simulink model "RefBlocks"  (R2020b)
settings: Solver=VariableStepAuto  StartTime=0.0  StopTime=10.0  RelTol=1e-3
values from neighbouring files (symbols this model uses):
  accel = 10000    [init_sim.m]
  Bm = 0    [init_sim.m]
  Ctrl_type = 3    [init_sim.m]
  dT = motorModel.SyreDrive.Converter.dT * 1e-6    [init_sim.m]
  expC = motorModel.IronPMLossMap_dq.expC    [init_sim.m]
  expH = motorModel.IronPMLossMap_dq.expH    [init_sim.m]
  expPM = motorModel.IronPMLossMap_dq.expPM    [init_sim.m]
  fD_pu_norm = motorModel.FluxMapInv_dq.fD_pu_norm    [init_sim.m]
  fD_vct_max = motorModel.FluxMapInv_dq.fD_vct_max    [init_sim.m]
  fD_vct_ref = motorModel.FluxMapInv_dq.fD_vct_ref    [init_sim.m]
  Fm = interp2(Idd,Iqq,Fdd,0,0)    [init_sim.m]
  fQ_pu_norm = motorModel.FluxMapInv_dq.fQ_pu_norm    [init_sim.m]
  fQ_vct_max = motorModel.FluxMapInv_dq.fQ_vct_max    [init_sim.m]
  fQ_vct_ref = motorModel.FluxMapInv_dq.fQ_vct_ref    [init_sim.m]
  Id_dqt = interpn(motorModel.FluxMapInv_dqt.dataF.Fd,motorModel.FluxMapInv_dqt.dataF.Fq,motorModel.FluxMapInv_dqt.dataF.th,motorModel.FluxMapInv_dqt.dataF.Id,Fd_dqt,Fq_dqt,th_dqt,'cubic')    [init_sim.m]
  Id_fe = motorModel.IronPMLossMap_dq.Id    [init_sim.m]
  id_MTPA = interp1(abs(MTPA.id+1i*MTPA.iq),MTPA.id,i0)    [init_sim.m]
  iD_pu_norm = motorModel.FluxMapInv_dq.iD_pu_norm    [init_sim.m]
  Iq_dqt = interpn(motorModel.FluxMapInv_dqt.dataF.Fd,motorModel.FluxMapInv_dqt.dataF.Fq,motorModel.FluxMapInv_dqt.dataF.th,motorModel.FluxMapInv_dqt.dataF.Iq,Fd_dqt,Fq_dqt,th_dqt,'cubic')    [init_sim.m]
  Iq_fe = motorModel.IronPMLossMap_dq.Iq    [init_sim.m]
  iq_MTPA = interp1(abs(MTPA.id+1i*MTPA.iq),MTPA.iq,i0)    [init_sim.m]
  iQ_pu_norm = motorModel.FluxMapInv_dq.iQ_pu_norm    [init_sim.m]
  IronLoss = 1    [init_sim.m]
  J = motorModel.data.J    [init_sim.m]
  L_sigma = Lq_inic*0.1    [init_sim.m]
  n0 = motorModel.IronPMLossMap_dq.n0    [init_sim.m]
  n_phase = n_set*3    [init_sim.m]
  p = motorModel.data.p    [init_sim.m]
  Pfe_c = motorModel.IronPMLossMap_dq.Pfes_c + motorModel.IronPMLossMap_dq.Pfer_c    [init_sim.m]
  Pfe_h = motorModel.IronPMLossMap_dq.Pfes_h + motorModel.IronPMLossMap_dq.Pfer_h    [init_sim.m]
  Ppm = motorModel.IronPMLossMap_dq.Ppm    [init_sim.m]
  Quad_Maps = 2    [init_sim.m]
  T_dqt = interpn(motorModel.FluxMapInv_dqt.dataF.Fd,motorModel.FluxMapInv_dqt.dataF.Fq,motorModel.FluxMapInv_dqt.dataF.th,motorModel.FluxMapInv_dqt.dataF.T,Fd_dqt,Fq_dqt,th_dqt,'cubic')    [init_sim.m]
  Tf = 0    [init_sim.m]
  th0 = 0    [init_sim.m]
  th_max = max(motorModel.FluxMapInv_dqt.dataF.th,[],'all')    [init_sim.m]
  th_min = min(motorModel.FluxMapInv_dqt.dataF.th,[],'all')    [init_sim.m]
  Ts = 1/motorModel.SyreDrive.Converter.fPWM    [init_sim.m]
  Tv = 0    [init_sim.m]
  VDC = motorModel.data.Vdc    [init_sim.m]
undefined symbols (not defined in the file or in its folder): magnitude, sigbuilder_block, T0
libraries: nesl_utility x8, simulink x4, ee_lib x4, fl_lib x2
(part 1 of 2)
settings Model: Creator=andyb  LastModifiedBy=andyb
settings DebuggingCC: UnconnectedInputMsg=none  UnconnectedOutputMsg=none  UnconnectedLineMsg=none
settings ModelReferenceCC: EnableRefExpFcnMdlSchedulingChecks=off

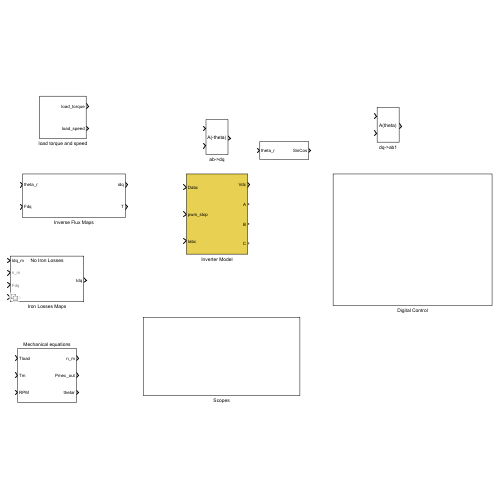
[thumbnail: Simulink's stored preview of the top-level diagram]
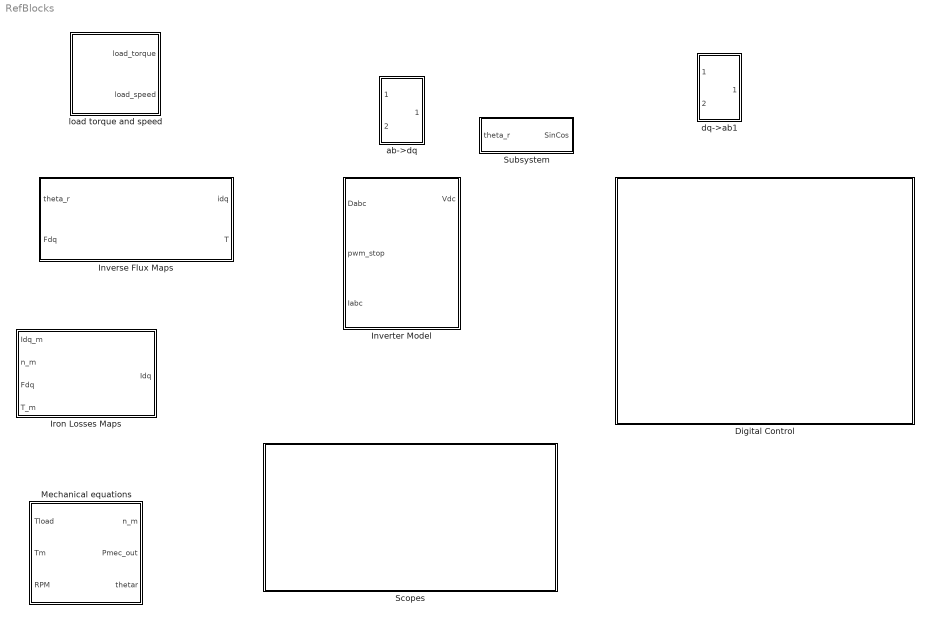
== system RefBlocks ==
  Digital Control : Subsystem
  Inverse Flux Maps : Subsystem
  Inverter Model : Subsystem
  Iron Losses Maps : Subsystem  Variant=on
  Mechanical equations : Subsystem
  Scopes : Subsystem
  Subsystem : Subsystem
  ab->dq : Subsystem
      mask Display: disp('A(-theta)')
  dq->ab1 : Subsystem
      mask Display: disp('A(theta)')
  load torque and speed : Subsystem

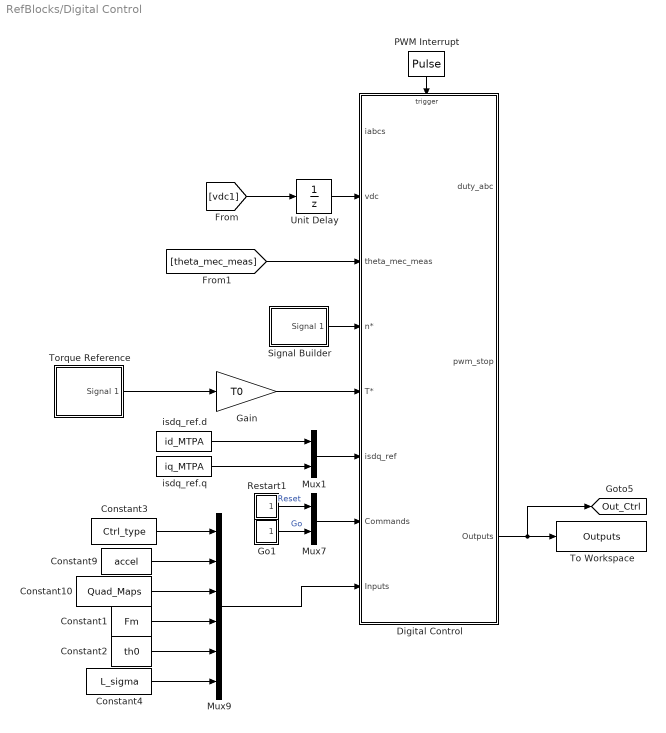
== system RefBlocks/Digital Control ==
  Constant1 : Constant  Value=Fm
  Constant10 : Constant  Value=Quad_Maps
  Constant2 : Constant  Value=th0
  Constant3 : Constant  Value=Ctrl_type
  Constant4 : Constant  Value=L_sigma
  Constant9 : Constant  Value=accel
  Digital Control : Subsystem  TreatAsAtomicUnit=on
  Gain : Gain  Gain=T0
  Go1 : Subsystem
  Mux1 : Mux  Inputs=2
  Mux7 : Mux  Inputs=2
  Mux9 : Mux  Inputs=6
  PWM Interrupt : DiscretePulseGenerator  PulseType=Time based  Period=Ts  PulseWidth=50
  Restart1 : Subsystem
  Signal Builder : Subsystem  Tag=STV Subsys  LoadFcn=sigbuilder_block('load');  StartFcn=sigbuilder_block('start');  StopFcn=sigbuilder_block('stop');  ClipboardFcn=sigbuilder_block('clipboard');  mask(Sigbuilder block){tuvar=[0:10]}
      mask help: Simulink:masks:SigbuilderBlock_MD
      mask init:
      | if ~strcmp(get_param(bdroot(gcbh),'SimulationStatus'),'stopped') tuvar = sigbuilder_block('maskInit'); end
      settings: CopyFcn=sigbuilder_block('copy');  DeleteFcn=sigbuilder_block('delete');  ModelCloseFcn=sigbuilder_block('modelClose');  PreSaveFcn=sigbuilder_block('preSave');  PauseFcn=sigbuilder_block('pause');  ContinueFcn=sigbuilder_block('continue');  NameChangeFcn=sigbuilder_block('namechange');  OpenFcn=sigbuilder_block('open',[163.8 121.8 550.2 399.6 ]);  CloseFcn=sigbuilder_block('close');
      mask Display: plot(0, 0, 100, 100,[2, 2, 32, 32, 2], [68, 8, 8, 68, 68],[32, 2], [38, 38], [32, 19, 2],[53, 60, 44], [32, 17, 17, 2],[16, 16, 31, 31]);txt = getActiveGroup(gcbh);text(2, 100, txt,'verticalAlignment', 'top');
  To Workspace : ToWorkspace  VariableName=Outputs  SaveFormat=Timeseries  SampleTime=-1
  Torque Reference : Subsystem  Tag=STV Subsys  LoadFcn=sigbuilder_block('load');  StartFcn=sigbuilder_block('start');  StopFcn=sigbuilder_block('stop');  ClipboardFcn=sigbuilder_block('clipboard');  mask(Sigbuilder block){tuvar=[0:10]}
      mask help: Simulink:masks:SigbuilderBlock_MD
      mask init:
      | if ~strcmp(get_param(bdroot(gcbh),'SimulationStatus'),'stopped') tuvar = sigbuilder_block('maskInit'); end
      settings: CopyFcn=sigbuilder_block('copy');  DeleteFcn=sigbuilder_block('delete');  ModelCloseFcn=sigbuilder_block('modelClose');  PreSaveFcn=sigbuilder_block('preSave');  PauseFcn=sigbuilder_block('pause');  ContinueFcn=sigbuilder_block('continue');  NameChangeFcn=sigbuilder_block('namechange');  OpenFcn=sigbuilder_block('open',[596.4 129.6 550.2 321.6 ]);  CloseFcn=sigbuilder_block('close');
      mask Display: plot(0, 0, 100, 100,[2, 2, 32, 32, 2], [68, 8, 8, 68, 68],[32, 2], [38, 38], [32, 19, 2],[53, 60, 44], [32, 17, 17, 2],[16, 16, 31, 31]);txt = getActiveGroup(gcbh);text(2, 100, txt,'verticalAlignment', 'top');
  Unit Delay : UnitDelay  SampleTime=-1  HasFrameUpgradeWarning=on
  isdq_ref.d : Constant  Value=id_MTPA
  isdq_ref.q : Constant  Value=iq_MTPA
  tag scope: Out_Ctrl=global
  wires:
  isdq_ref.d/1 -> Mux1/1
  Restart1/1(Res) -> Mux7/1  "Reset"
  Mux9/1 -> Digital Control/8(Inputs)
  PWM Interrupt/1 -> Digital Control/Trigger
  Mux7/1 -> Digital Control/7(Commands)
  Unit Delay/1 -> Digital Control/2(vdc)
  Gain/1 -> Digital Control/5(T*)
  Go1/1(Go) -> Mux7/2  "Go"
  Digital Control/3(Outputs) -> [Out_Ctrl], To Workspace/1
  Constant3/1 -> Mux9/1
  Mux1/1 -> Digital Control/6(isdq_ref)
  Torque Reference/1(Signal 1) -> Gain/1
  Signal Builder/1(Signal 1) -> Digital Control/4(n*)
  isdq_ref.q/1 -> Mux1/2
  [vdc1] -> Unit Delay/1
  [theta_mec_meas] -> Digital Control/3(theta_mec_meas)
  Constant9/1 -> Mux9/2
  Constant10/1 -> Mux9/3
  Constant1/1 -> Mux9/4
  Constant2/1 -> Mux9/5
  Constant4/1 -> Mux9/6

== system RefBlocks/Inverse Flux Maps ==
  theta_r : Inport
  Fdq : Inport  Port=2
  Gain : Gain  Gain=p
  "Inverse Flux Maps " : Subsystem  Variant=on
  idq : Outport
  T : Outport  Port=2
  wires:
  "Inverse Flux Maps "/2(T) -> T/1
  "Inverse Flux Maps "/1(idq) -> idq/1
  theta_r/1 -> Gain/1
  Fdq/1 -> "Inverse Flux Maps "/1(Fdq)
  Gain/1 -> "Inverse Flux Maps "/2(theta_elt)

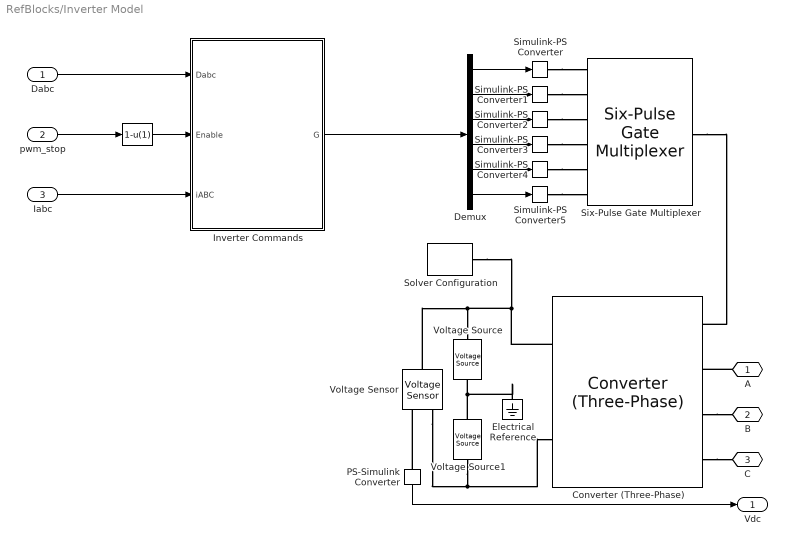
== system RefBlocks/Inverter Model ==
  Dabc : Inport
  pwm_stop : Inport  Port=2
  Iabc : Inport  Port=3
  " " : Fcn  Expr=1-u(1)
  Converter (Three-Phase) : ee_lib/Semiconductors & Converters/Converters/Converter (Three-Phase)  port_option=ee.enum.threePhasePort.expanded  device_type=ee.enum.converters.switchingdevice.ideal  K=0  Vf=0.001 V  Ron=Rd Ohm  Rds=0.001 Ohm  Goff=1e-4 1/Ohm  Vgt=1 V  Vgt_off=-1 V  Ih=1 A  Vth=0.001 V  diode_param=ee.enum.converters.protectiondiode.nodynamics  diode_Vf=0.8 V  diode_Ron=1e-4 Ohm  diode_Goff=1e-5 1/Ohm  diode_C=50 nF  diode_iRM=-235 A  diode_iF=300 A  diode_idot=-50 A/us  diode_trr_param=ee.enum.converters.diodetrr.trr_factor  diode_trr_factor=3  diode_trr=15 us  diode_Qrr=1500 s*uA  snubber_type=ee.enum.converters.snubber.exclude  Cs=1e-7 F  Rs=0.1 Ohm
      settings: InternalSimscapePortConfiguration="{\"Bottom\":[],\"Left\":[{\"id\":\"G\",\"label\":\"G\",\"type\":\"foundation.electrical.twelve_phase\"},{\"id\":\"a\",\"label\":\"a\",\"type\":\"foundation.electrical.electrical\"},{\"id\":\"b\",\"label\":\"b\",\"type\":\"foundation.electrical.electrical\"},{\"id\":\"c\",\"label\":\"c\",\"type\":\"foundation.electrical.electrical\"}],\"Right\":[{\"id\":\"p\",\"label\":\"+\",\"type\":\"foundation.electrical.electrical\"},{\"id\":\"n\",\"label\":\"-\",\"type\":\"foundation.electrical.electrical\"}],\"Top\":[]}"
  Demux : Demux  Outputs=6
  Electrical Reference : fl_lib/Electrical/Electrical Elements/Electrical Reference
  Inverter Commands : Subsystem  Variant=on
  PS-Simulink Converter : nesl_utility/PS-Simulink Converter  PhysicalDomain=network_engine_domain  SubClassName=ps_output  LeftPortType=input  RightPortType=output  PseudoPeriodic=off  Frequencies=[]  VectorFormat=1-D array  Unit=inherit  AffineConversion=off
  Simulink-PS Converter{,1..5} (6 alike) : nesl_utility/Simulink-PS Converter  PhysicalDomain=network_engine_domain  SubClassName=ps_input  LeftPortType=input  RightPortType=output  PseudoPeriodic=off  Frequencies=[]  NoiseDistribution=none  NoiseParameters=[]  Unit=1  AffineConversion=off  FilteringAndDerivatives=provide  SimscapeFilterOrder=1  InputFilterTimeConstant=0.001  UdotUserProvided=0
  Six-Pulse Gate Multiplexer : ee_lib/Semiconductors & Converters/Converters/Six-Pulse Gate Multiplexer  port_option=ee.enum.controlport.ps
  Solver Configuration : nesl_utility/Solver Configuration  PhysicalDomain=network_engine_domain  SubClassName=solver  LeftPortType=input  RightPortType=generic  Tones=[]  Harmonics=[]  SimulateNoise=off  Profile=off  UseLocalSampling=off  EnableSwitchedLinearOptims=on  FrequencyDomain=off  UseCCode=off  RelTol=0.001  AbsTol=1e-06  MinStep=1e-09  ToWorkspace=off  RevertToSquareIcSolve=off  NumHomotopyIterations=100  PhasorMode=off  PhasorModeNumHarmonics=1  ConsistencySolver=NEWTON_FTOL  IndexReductionMethod=DerivativeReplacement  DoDC=off  ResidualTolerance=1e-09  ConsistencyTolSource=GLOBAL  ConsistencyAbsTol=0.001  ConsistencyRelTol=0.001  ConsistencyTolFactor=0.001  UseLocalSolver=off  LocalSolverChoice=NE_BACKWARD_EULER_ADVANCER  ResolveIndetEquations=on  FunctionEvalNumThread=1  LocalSolverSampleTime=Ts  DoFixedCost=off  MaxNonlinIter=3  MaxModeIter=2  ComputeImpulses=off  ImpulseIterations=2  LinearAlgebra=auto  LinearAlgebraNumThread=0  EquationFormulation=NE_TIME_EF  DelaysMemoryBudget=1024  AutomaticFiltering=on  FilteringTimeConstant=0.001  PartitionStorageMethod=AS_NEEDED  PartitionMemoryBudget=1024  PartitionMethod=ROBUST  MultibodyUseLocalSolver=off  MultibodyLocalSolverChoice=ODE1  MultibodyLocalSolverSampleTime=0.001
  Voltage Sensor : fl_lib/Electrical/Electrical Sensors/Voltage Sensor
  Voltage Source : ee_lib/Sources/Voltage Source  dc_voltage=0.5*VDC V  ac_voltage=0 V  ac_shift=0 rad  ac_frequency=60 Hz  noise_mode=0  PSD=0 V^2/Hz  sample_time=1e-3 s  repeatability=1  user_seed=0  auto_seed=2348838240  i_specify=off  i_priority=None  i=0 A  i_nominal_specify=off  i_nominal_unit=A  i_nominal_value=1  v_specify=off  v_priority=None  v=0 V  v_nominal_specify=off  v_nominal_unit=V  v_nominal_value=1
  Voltage Source1 : ee_lib/Sources/Voltage Source  dc_voltage=0.5*VDC V  ac_voltage=0 V  ac_shift=0 rad  ac_frequency=60 Hz  noise_mode=0  PSD=0 V^2/Hz  sample_time=1e-3 s  repeatability=1  user_seed=0  auto_seed=4112460543  i_specify=off  i_priority=None  i=0 A  i_nominal_specify=off  i_nominal_unit=A  i_nominal_value=1  v_specify=off  v_priority=None  v=0 V  v_nominal_specify=off  v_nominal_unit=V  v_nominal_value=1
  A : PMIOPort  Side=Right
  B : PMIOPort  Port=2  Side=Right
  C : PMIOPort  Port=3  Side=Right
  Vdc : Outport
  wires:
  Iabc/1 -> Inverter Commands/3(iABC)
  Demux/3 -> Simulink-PS Converter2/1
  Demux/4 -> Simulink-PS Converter3/1
  Demux/5 -> Simulink-PS Converter4/1
  Demux/6 -> Simulink-PS Converter5/1
  Demux/1 -> Simulink-PS Converter/1
  Demux/2 -> Simulink-PS Converter1/1
  pwm_stop/1 -> " "/1
  " "/1 -> Inverter Commands/2(Enable)
  PS-Simulink Converter/1 -> Vdc/1
  Dabc/1 -> Inverter Commands/1(Dabc)
  Inverter Commands/1(G) -> Demux/1
  connections:
  Simulink-PS Converter/RConn1 -- Six-Pulse Gate Multiplexer/LConn1
  Simulink-PS Converter3/RConn1 -- Six-Pulse Gate Multiplexer/LConn4
  Solver Configuration/RConn1 -- Converter (Three-Phase)/RConn1 -- Voltage Sensor/LConn1 -- Voltage Source/LConn1
  Simulink-PS Converter4/RConn1 -- Six-Pulse Gate Multiplexer/LConn5
  Simulink-PS Converter2/RConn1 -- Six-Pulse Gate Multiplexer/LConn3
  Simulink-PS Converter1/RConn1 -- Six-Pulse Gate Multiplexer/LConn2
  Simulink-PS Converter5/RConn1 -- Six-Pulse Gate Multiplexer/LConn6
  Voltage Source1/RConn1 -- Converter (Three-Phase)/RConn2 -- Voltage Sensor/RConn2
  Voltage Source/RConn1 -- Voltage Source1/LConn1 -- Electrical Reference/LConn1
  Six-Pulse Gate Multiplexer/RConn1 -- Converter (Three-Phase)/LConn1
  A/RConn1 -- Converter (Three-Phase)/LConn2
  Converter (Three-Phase)/LConn3 -- B/RConn1
  Converter (Three-Phase)/LConn4 -- C/RConn1
  PS-Simulink Converter/LConn1 -- Voltage Sensor/RConn1

== system RefBlocks/Iron Losses Maps ==
  note: 1) Add Subsystem or Model blocks as valid variant choices.
      | 2) You cannot connect blocks at this level. At simulation, connectivity is automatically
      | determined, based on the active variant and port name matching.
  Idq_m : Inport
  n_m : Inport  Port=2
  Fdq : Inport  Port=3
  T_m : Inport  Port=4
  Iron Losses : Subsystem  VariantControl=IronLoss==1
  No Iron Losses : Subsystem  VariantControl=IronLoss==0
  Idq : Outport

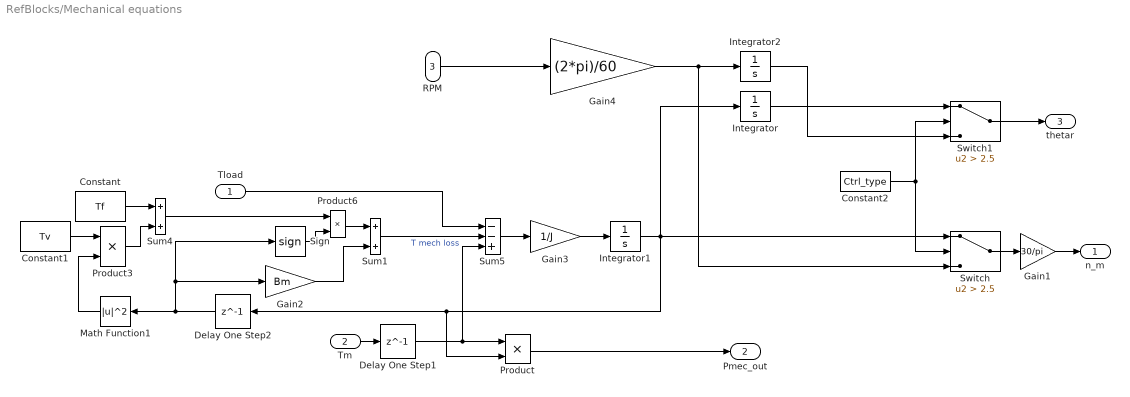
== system RefBlocks/Mechanical equations ==
  Tload : Inport
  Tm : Inport  Port=2
  RPM : Inport  Port=3
  Constant : Constant  Value=Tf
  Constant1 : Constant  Value=Tv
  Constant2 : Constant  Value=Ctrl_type
  Delay One Step1 : Delay  DelayLength=1
  Delay One Step2 : Delay  DelayLength=1
  Gain1 : Gain  Gain=30/pi
  Gain2 : Gain  Gain=Bm  SaturateOnIntegerOverflow=on  OutDataTypeStr=Inherit: Same as input  ParamDataTypeStr=Inherit: Same as input
  Gain3 : Gain  Gain=1/J  SaturateOnIntegerOverflow=on  OutDataTypeStr=Inherit: Same as input  ParamDataTypeStr=Inherit: Same as input
  Gain4 : Gain  Gain=(2*pi)/60
  Integrator : Integrator  InitialCondition=th0  WrapState=on  WrappedStateUpperValue=2*pi  WrappedStateLowerValue=0
  Integrator1 : Integrator
  Integrator2 : Integrator  InitialCondition=th0  WrapState=on  WrappedStateUpperValue=2*pi  WrappedStateLowerValue=0
  Math Function1 : Math  Operator=magnitude^2  SignedPower=on  SaturateOnIntegerOverflow=on
  Product : Product  SaturateOnIntegerOverflow=on  OutDataTypeStr=Inherit: Same as first input
  Product3 : Product  SaturateOnIntegerOverflow=on  OutDataTypeStr=Inherit: Same as first input
  Product6 : Product  SaturateOnIntegerOverflow=on  OutDataTypeStr=Inherit: Same as first input
  Sign : Signum  ZeroCross=off
  Sum1 : Sum  SaturateOnIntegerOverflow=on  OutDataTypeStr=Inherit: Same as first input
  Sum4 : Sum  SaturateOnIntegerOverflow=on  OutDataTypeStr=Inherit: Same as first input
  Sum5 : Sum  Inputs=--+  SaturateOnIntegerOverflow=on  OutDataTypeStr=Inherit: Same as first input
  Switch : Switch  Criteria=u2 > Threshold  Threshold=2.5
  Switch1 : Switch  Criteria=u2 > Threshold  Threshold=2.5
  n_m : Outport
  Pmec_out : Outport  Port=2  VectorParamsAs1DForOutWhenUnconnected=off
  thetar : Outport  Port=3
  wires:
  Gain3/1 -> Integrator1/1
  Gain2/1 -> Sum1/2
  Delay One Step2/1 -> Math Function1/1, Sign/1, Gain2/1
  Product6/1 -> Sum1/1
  Sum1/1 -> Sum5/2  "T mech loss"
  Tm/1 -> Delay One Step1/1
  Product/1 -> Pmec_out/1
  Tload/1 -> Sum5/1
  Math Function1/1 -> Product3/2
  Constant1/1 -> Product3/1
  Product3/1 -> Sum4/2
  Constant/1 -> Sum4/1
  Sum5/1 -> Gain3/1
  Sign/1 -> Product6/2
  Sum4/1 -> Product6/1
  Integrator2/1 -> Switch1/3
  Integrator/1 -> Switch1/1
  Switch1/1 -> thetar/1
  Switch/1 -> Gain1/1
  Integrator1/1 -> Integrator/1, Switch/1, Delay One Step2/1, Product/2
  Gain4/1 -> Switch/3, Integrator2/1
  Constant2/1 -> Switch/2, Switch1/2
  RPM/1 -> Gain4/1
  Delay One Step1/1 -> Sum5/3, Product/1
  Gain1/1 -> n_m/1

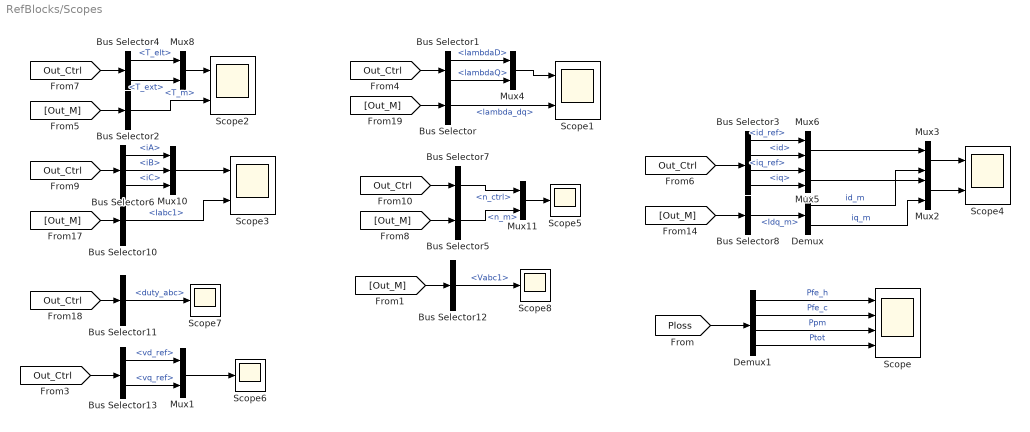
== system RefBlocks/Scopes ==
  Bus Selector : BusSelector  OutputSignals=lambda_dq
  Bus Selector1 : BusSelector  OutputSignals=lambdaD,lambdaQ
  Bus Selector10 : BusSelector  OutputSignals=Iabc1
  Bus Selector11 : BusSelector  OutputSignals=duty_abc
  Bus Selector12 : BusSelector  OutputSignals=Vabc1
  Bus Selector13 : BusSelector  OutputSignals=vd_ref,vq_ref
  Bus Selector2 : BusSelector  OutputSignals=T_m
  Bus Selector3 : BusSelector  OutputSignals=id_ref,id,iq_ref,iq
  Bus Selector4 : BusSelector  OutputSignals=T_elt,T_ext
  Bus Selector5 : BusSelector  OutputSignals=n_m
  Bus Selector6 : BusSelector  OutputSignals=iA,iB,iC
  Bus Selector7 : BusSelector  OutputSignals=n_ctrl
  Bus Selector8 : BusSelector  OutputSignals=Idq_m
  Demux : Demux  Outputs=2
  Demux1 : Demux
  Mux{1..6,8,11} (8 alike) : Mux  Inputs=2
  Mux10 : Mux  Inputs=3
  Scope : Scope  NumInputPorts=4
  Scope{1..4} (4 alike) : Scope  NumInputPorts=2
  Scope{5..8} (4 alike) : Scope
  wires:
  Bus Selector3/2 -> Mux6/2  "<id>"
  [Out_M] -> Bus Selector2/1
  Mux4/1 -> Scope1/1
  Bus Selector/1 -> Scope1/2  "<lambda_dq>"
  Bus Selector7/1 -> Mux11/1  "<n_ctrl>"
  Bus Selector1/2 -> Mux4/2  "<lambdaQ>"
  Bus Selector3/3 -> Mux5/1  "<iq_ref>"
  Bus Selector3/4 -> Mux5/2  "<iq>"
  Bus Selector4/1 -> Mux8/1  "<T_elt>"
  Mux6/1 -> Mux3/1
  Demux/1 -> Mux3/2  "id_m"
  [Out_M] -> Bus Selector5/1
  Bus Selector1/1 -> Mux4/1  "<lambdaD>"
  [Out_Ctrl] -> Bus Selector1/1
  [Out_Ctrl] -> Bus Selector4/1
  Mux5/1 -> Mux2/1
  [Out_Ctrl] -> Bus Selector7/1
  Bus Selector5/1 -> Mux11/2  "<n_m>"
  [Out_M] -> Bus Selector8/1
  Bus Selector3/1 -> Mux6/1  "<id_ref>"
  [Out_Ctrl] -> Bus Selector3/1
  Mux8/1 -> Scope2/1
  Bus Selector8/1 -> Demux/1  "<Idq_m>"
  Demux/2 -> Mux2/2  "iq_m"
  Bus Selector11/1 -> Scope7/1  "<duty_abc>"
  Mux3/1 -> Scope4/1
  [Out_Ctrl] -> Bus Selector11/1
  Mux2/1 -> Scope4/2
  [Out_M] -> Bus Selector/1
  Mux11/1 -> Scope5/1
  Demux1/1 -> Scope/1  "Pfe_h"
  Demux1/2 -> Scope/2  "Pfe_c"
  Demux1/4 -> Scope/4  "Ptot"
  Demux1/3 -> Scope/3  "Ppm"
  Bus Selector2/1 -> Scope2/2  "<T_m>"
  Bus Selector4/2 -> Mux8/2  "<T_ext>"
  [Out_Ctrl] -> Bus Selector13/1
  Mux1/1 -> Scope6/1
  Bus Selector13/1 -> Mux1/1  "<vd_ref>"
  Bus Selector13/2 -> Mux1/2  "<vq_ref>"
  [Ploss] -> Demux1/1
  Bus Selector6/1 -> Mux10/1  "<iA>"
  Mux10/1 -> Scope3/1
  Bus Selector10/1 -> Scope3/2  "<Iabc1>"
  Bus Selector6/2 -> Mux10/2  "<iB>"
  Bus Selector6/3 -> Mux10/3  "<iC>"
  [Out_Ctrl] -> Bus Selector6/1
  [Out_M] -> Bus Selector10/1
  [Out_M] -> Bus Selector12/1
  Bus Selector12/1 -> Scope8/1  "<Vabc1>"

== system RefBlocks/Subsystem ==
  theta_r : Inport
  Gain1 : Gain  Gain=p
  Mux3 : Mux  Inputs=2
  Scope : Scope
  Scope1 : Scope
  Sin : Trigonometry
  Sin1 : Trigonometry  Operator=cos
  SinCos : Outport
  wires:
  Sin1/1 -> Mux3/2
  Sin/1 -> Mux3/1
  Mux3/1 -> Scope/1, SinCos/1
  Gain1/1 -> Scope1/1, Sin/1, Sin1/1
  theta_r/1 -> Gain1/1

== system RefBlocks/ab->dq ==
  X_ab : Inport
  sin,cos : Inport  Port=2
  Demux : Demux  Outputs=2
  Demux1 : Demux  Outputs=2
  Mux : Mux  Commented=on  Inputs=2
  Mux1 : Mux  Commented=on  Inputs=2
  Mux2 : Mux  Inputs=2
  Product{,1..3} (4 alike) : Product
  Subtract : Sum
  Subtract1 : Sum  Inputs=-+
  X_d : Fcn  Commented=on  Expr=u(1)*u(4) + u(2)*u(3)
  X_q : Fcn  Commented=on  Expr=- u(1)*u(3) + u(2)*u(4)
  X_dq : Outport  InitialOutput=0
  wires:
  X_q/1 -> Mux1/2
  X_d/1 -> Mux1/1
  Mux/1 -> X_q/1, X_d/1
  Demux1/2 -> Product1/2, Product/2
  Demux/2 -> Product1/1, Product2/1
  Demux1/1 -> Product3/2, Product2/2
  Product/1 -> Subtract/1
  Product2/1 -> Subtract/2
  Demux/1 -> Product3/1, Product/1
  Product3/1 -> Subtract1/1
  Product1/1 -> Subtract1/2
  Subtract/1 -> Mux2/1
  Subtract1/1 -> Mux2/2
  X_ab/1 -> Demux/1
  sin,cos/1 -> Demux1/1
  Mux2/1 -> X_dq/1

== system RefBlocks/dq->ab1 ==
  X_ab : Inport
  sin,cos : Inport  Port=2
  Demux : Demux  Outputs=2
  Demux1 : Demux  Outputs=2
  Mux : Mux  Inputs=2
  Mux2 : Mux  Commented=on  Inputs=2
  Mux3 : Mux  Commented=on  Inputs=2
  Product{,1..3} (4 alike) : Product
  Subtract : Sum  Inputs=+-
  Subtract1 : Sum
  X_d1 : Fcn  Commented=on  Expr=u(1)*u(4) - u(2)*u(3)
  X_q1 : Fcn  Commented=on  Expr=u(1)*u(3) + u(2)*u(4)
  X_dq : Outport  InitialOutput=0
  wires:
  Mux3/1 -> X_d1/1, X_q1/1
  X_d1/1 -> Mux2/1
  X_q1/1 -> Mux2/2
  Demux/1 -> Product2/1, Product/1
  Demux1/2 -> Product3/2, Product/2
  Product1/1 -> Subtract/2
  Product/1 -> Subtract/1
  Demux/2 -> Product3/1, Product1/1
  Demux1/1 -> Product2/2, Product1/2
  Product2/1 -> Subtract1/1
  Product3/1 -> Subtract1/2
  Subtract/1 -> Mux/1
  Subtract1/1 -> Mux/2
  X_ab/1 -> Demux/1
  sin,cos/1 -> Demux1/1
  Mux/1 -> X_dq/1

== system RefBlocks/load torque and speed ==
  Gain3 : Gain  Gain=n0
  Gain4 : Gain  Gain=T0
  load speed : Subsystem  Tag=STV Subsys  LoadFcn=sigbuilder_block('load');  StartFcn=sigbuilder_block('start');  StopFcn=sigbuilder_block('stop');  ClipboardFcn=sigbuilder_block('clipboard');  mask(Sigbuilder block){tuvar=[0:10]}
      mask help: Simulink:masks:SigbuilderBlock_MD
      mask init:
      | if ~strcmp(get_param(bdroot(gcbh),'SimulationStatus'),'stopped') tuvar = sigbuilder_block('maskInit'); end
      settings: CopyFcn=sigbuilder_block('copy');  DeleteFcn=sigbuilder_block('delete');  ModelCloseFcn=sigbuilder_block('modelClose');  PreSaveFcn=sigbuilder_block('preSave');  PauseFcn=sigbuilder_block('pause');  ContinueFcn=sigbuilder_block('continue');  NameChangeFcn=sigbuilder_block('namechange');  OpenFcn=sigbuilder_block('open',[1960.8 11.4 550.2 315.6 ]);  CloseFcn=sigbuilder_block('close');
      mask Display: plot(0, 0, 100, 100,[2, 2, 32, 32, 2], [68, 8, 8, 68, 68],[32, 2], [38, 38], [32, 19, 2],[53, 60, 44], [32, 17, 17, 2],[16, 16, 31, 31]);txt = getActiveGroup(gcbh);text(2, 100, txt,'verticalAlignment', 'top');
  load torque : Subsystem  Tag=STV Subsys  LoadFcn=sigbuilder_block('load');  StartFcn=sigbuilder_block('start');  StopFcn=sigbuilder_block('stop');  ClipboardFcn=sigbuilder_block('clipboard');  mask(Sigbuilder block){tuvar=[0:10]}
      mask help: Simulink:masks:SigbuilderBlock_MD
      mask init:
      | if ~strcmp(get_param(bdroot(gcbh),'SimulationStatus'),'stopped') tuvar = sigbuilder_block('maskInit'); end
      settings: CopyFcn=sigbuilder_block('copy');  DeleteFcn=sigbuilder_block('delete');  ModelCloseFcn=sigbuilder_block('modelClose');  PreSaveFcn=sigbuilder_block('preSave');  PauseFcn=sigbuilder_block('pause');  ContinueFcn=sigbuilder_block('continue');  NameChangeFcn=sigbuilder_block('namechange');  OpenFcn=sigbuilder_block('open',[246.6 156.6 550.2 360.6 ]);  CloseFcn=sigbuilder_block('close');
      mask Display: plot(0, 0, 100, 100,[2, 2, 32, 32, 2], [68, 8, 8, 68, 68],[32, 2], [38, 38], [32, 19, 2],[53, 60, 44], [32, 17, 17, 2],[16, 16, 31, 31]);txt = getActiveGroup(gcbh);text(2, 100, txt,'verticalAlignment', 'top');
  load_torque : Outport
  load_speed : Outport  Port=2
  tag scope: T_load=global
  wires:
  load speed/1(Signal 1) -> Gain3/1
  load torque/1(Signal 1) -> Gain4/1
  Gain4/1 -> load_torque/1, [T_load]
  Gain3/1 -> load_speed/1

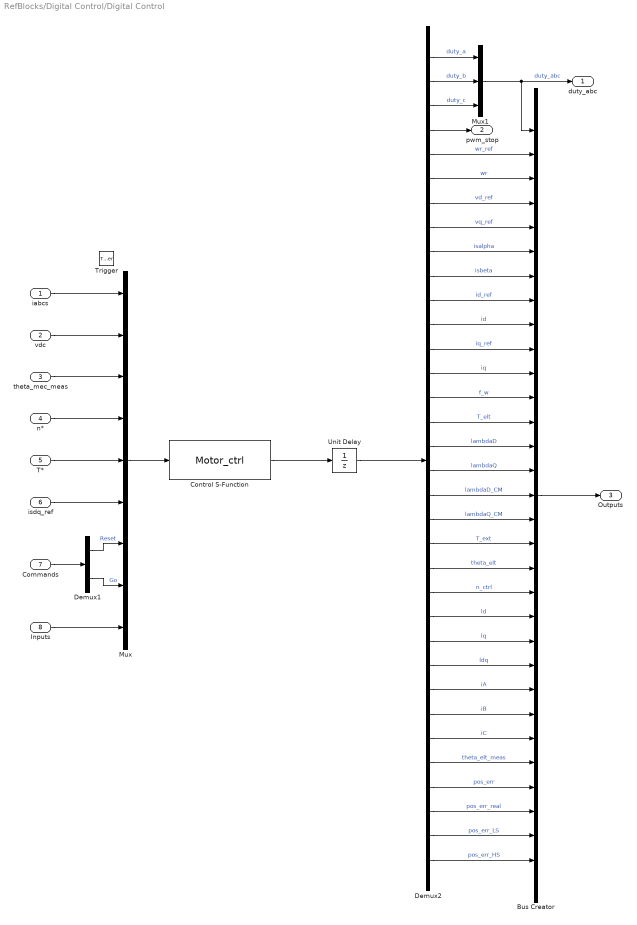
== system RefBlocks/Digital Control/Digital Control ==
  iabcs : Inport
  vdc : Inport  Port=2
  theta_mec_meas : Inport  Port=3
  n* : Inport  Port=4
  T* : Inport  Port=5
  isdq_ref : Inport  Port=6
  Commands : Inport  Port=7
  Inputs : Inport  Port=8
  Trigger : TriggerPort  VariantControl=(inherit)
  Bus Creator : BusCreator  Inputs=31
  Control S-Function : S-Function  FunctionName=Motor_ctrl  SFunctionDeploymentMode=off  EnableBusSupport=off
  Demux1 : Demux  Outputs=2
  Demux2 : Demux  Outputs=34
  Mux : Mux  Inputs=9
  Mux1 : Mux  Inputs=3
  Unit Delay : UnitDelay  SampleTime=-1  HasFrameUpgradeWarning=on
  duty_abc : Outport
  pwm_stop : Outport  Port=2
  Outputs : Outport  Port=3
  wires:
  Mux/1 -> Control S-Function/1
  vdc/1 -> Mux/2
  theta_mec_meas/1 -> Mux/3
  Control S-Function/1 -> Unit Delay/1
  n*/1 -> Mux/4
  Mux1/1 -> duty_abc/1, Bus Creator/1  "duty_abc"
  Demux1/1 -> Mux/7  "Reset"
  Demux1/2 -> Mux/8  "Go"
  Commands/1 -> Demux1/1
  isdq_ref/1 -> Mux/6
  Unit Delay/1 -> Demux2/1
  Demux2/1 -> Mux1/1  "duty_a"
  Demux2/2 -> Mux1/2  "duty_b"
  Demux2/3 -> Mux1/3  "duty_c"
  Demux2/4 -> pwm_stop/1
  T*/1 -> Mux/5
  Inputs/1 -> Mux/9
  Bus Creator/1 -> Outputs/1
  Demux2/34 -> Bus Creator/31  "pos_err_HS"
  Demux2/33 -> Bus Creator/30  "pos_err_LS"
  Demux2/32 -> Bus Creator/29  "pos_err_real"
  Demux2/31 -> Bus Creator/28  "pos_err"
  Demux2/30 -> Bus Creator/27  "theta_elt_meas"
  Demux2/29 -> Bus Creator/26  "iC"
  Demux2/28 -> Bus Creator/25  "iB"
  Demux2/27 -> Bus Creator/24  "iA"
  Demux2/26 -> Bus Creator/23  "ldq"
  Demux2/25 -> Bus Creator/22  "lq"
  Demux2/24 -> Bus Creator/21  "ld"
  Demux2/23 -> Bus Creator/20  "n_ctrl"
  Demux2/22 -> Bus Creator/19  "theta_elt"
  Demux2/21 -> Bus Creator/18  "T_ext"
  Demux2/20 -> Bus Creator/17  "lambdaQ_CM"
  Demux2/18 -> Bus Creator/15  "lambdaQ"
  Demux2/19 -> Bus Creator/16  "lambdaD_CM"
  Demux2/17 -> Bus Creator/14  "lambdaD"
  Demux2/16 -> Bus Creator/13  "T_elt"
  Demux2/15 -> Bus Creator/12  "f_w"
  Demux2/14 -> Bus Creator/11  "iq"
  Demux2/13 -> Bus Creator/10  "iq_ref"
  Demux2/12 -> Bus Creator/9  "id"
  Demux2/11 -> Bus Creator/8  "id_ref"
  Demux2/10 -> Bus Creator/7  "isbeta"
  Demux2/9 -> Bus Creator/6  "isalpha"
  Demux2/8 -> Bus Creator/5  "vq_ref"
  Demux2/7 -> Bus Creator/4  "vd_ref"
  Demux2/6 -> Bus Creator/3  "wr"
  Demux2/5 -> Bus Creator/2  "wr_ref"
  iabcs/1 -> Mux/1

== system RefBlocks/Digital Control/Go1 ==
  Constant : Constant  Value=0
  GO1_Down : Step  Time=0.03+4*Ts  SampleTime=0
  GO1_Up : Step  Time=0.03  SampleTime=0
  GO2_Down : Step  Time=0.1+4*Ts  SampleTime=0
  GO2_Up : Step  Time=0.1  SampleTime=0
  Subtract : Sum  Inputs=++-+-
  Go : Outport
  wires:
  Subtract/1 -> Go/1
  Constant/1 -> Subtract/1
  GO1_Up/1 -> Subtract/2
  GO1_Down/1 -> Subtract/3
  GO2_Up/1 -> Subtract/4
  GO2_Down/1 -> Subtract/5

== system RefBlocks/Digital Control/Restart1 ==
  "DOWN " : Step  Time=10e-3+4*Ts  SampleTime=0
  Subtract : Sum  Inputs=+-
  "UP " : Step  Time=10e-3  SampleTime=0
  Res : Outport
  wires:
  "UP "/1 -> Subtract/1
  "DOWN "/1 -> Subtract/2
  Subtract/1 -> Res/1

== system RefBlocks/Digital Control/Signal Builder ==
  Demux : Demux  Tag=STV Demux  Outputs=1
      settings: DisplayOption=none
  FromWs : FromWorkspace  Tag=STV FromWs  VariableName=tuvar
      SigBuilderData=|
      | common.afterFinalStr = 'Extrapolate'
      | common.sampleTime = 0
      | dataSet.timeRange = [0 10]
      | dataSet.name = 'Group 1'
      | sbobj.Groups.Name = 'Group 1'
      | sbobj.Groups.Signals.Name = 'Signal 1'
      | sbobj.Groups.Signals.XData = [0 1.98 1.98 8 8 10]
      | sbobj.Groups.Signals.YData = [0 0 1500 1500 -1500 -1500]
  Signal 1 : Outport  Tag=STV Outport
  wires:
  Demux/1 -> Signal 1/1
  FromWs/1 -> Demux/1

== system RefBlocks/Digital Control/Torque Reference ==
  Demux : Demux  Tag=STV Demux  Outputs=1
      settings: DisplayOption=none
  FromWs : FromWorkspace  Tag=STV FromWs  VariableName=tuvar
      SigBuilderData=|
      | common.afterFinalStr = 'Extrapolate'
      | common.sampleTime = 0
      | dataSet.timeRange = [0 2]
      | dataSet.name = 'Group 1'
      | sbobj.Groups.Name = 'Group 1'
      | sbobj.Groups.Signals.Name = 'Signal 1'
      | sbobj.Groups.Signals.XData = [0 0.15 0.15 0.8 0.8 2]
      | sbobj.Groups.Signals.YData = [0 0 1 1 -1 -1]
      | sbobj.Groups.TimeRange = [0 2]
  Signal 1 : Outport  Tag=STV Outport
  wires:
  FromWs/1 -> Demux/1
  Demux/1 -> Signal 1/1

== system RefBlocks/Inverse Flux Maps/Inverse Flux Maps  ==
  note: 1) Add Subsystem or Model blocks as valid variant choices.
      | 2) You cannot connect blocks at this level. At simulation, connectivity is automatically
      | determined, based on the active variant and port name matching.
  Fdq : Inport
  theta_elt : Inport  Port=2
  2D LUT : Subsystem  VariantControl=FMapsModel==1
  3D LUTs : Subsystem  VariantControl=FMapsModel==-1
  idq : Outport
  T : Outport  Port=2

== system RefBlocks/Inverter Model/Inverter Commands ==
  note: 1) Add Subsystem or Model blocks as valid variant choices.
      | 2) You cannot connect blocks at this level. At simulation, connectivity is automatically
      | determined, based on the active variant and port name matching.
  Dabc : Inport
  Enable : Inport  Port=2
  iABC : Inport  Port=3
  Duty : Subsystem  VariantControl=InvModel==0
  PWM : Subsystem  VariantControl=InvModel==1
  G : Outport

== system RefBlocks/Iron Losses Maps/Iron Losses ==
  Idq_m : Inport
  n_m : Inport  Port=2
  Fdq : Inport  Port=3
  Demux1 : Demux  Outputs=2
  Demux2 : Demux  Outputs=2
  Demux3 : Demux  Outputs=2
  Iron loss Maps : Subsystem
  Mux2 : Mux  Inputs=2
  Scope6 : Scope  NumInputPorts=2
  Sum1 : Sum  Inputs=|++
  Sum2 : Sum  Inputs=|++
  Idq : Outport
  tag scope: Ploss=global
  wires:
  Demux1/2 -> Sum2/1
  Sum2/1 -> Mux2/2
  Sum1/1 -> Mux2/1
  Demux1/1 -> Sum1/1
  Demux2/1 -> Sum1/2
  Demux2/2 -> Sum2/2
  Mux2/1 -> Idq/1
  Idq_m/1 -> Demux1/1, Iron loss Maps/1(Idq_m)
  n_m/1 -> Iron loss Maps/2(n_m)
  Fdq/1 -> Iron loss Maps/3(Fdq)
  Demux3/2 -> Scope6/2  "Iq_fe"
  Iron loss Maps/1(Idq_fe) -> Demux3/1, Demux2/1
  Demux3/1 -> Scope6/1  "Id_fe"
  Iron loss Maps/2(Ploss) -> [Ploss]

== system RefBlocks/Iron Losses Maps/No Iron Losses ==
  Idq_m : Inport
  Idq : Outport
  wires:
  Idq_m/1 -> Idq/1

== system RefBlocks/load torque and speed/load speed ==
  Demux : Demux  Tag=STV Demux  Outputs=1
      settings: DisplayOption=none
  FromWs : FromWorkspace  Tag=STV FromWs  VariableName=tuvar
      SigBuilderData=|
      | common.afterFinalStr = 'Extrapolate'
      | common.sampleTime = 0
      | dataSet.timeRange = [0 2]
      | dataSet.name = 'Group 1'
      | sbobj.Groups.Name = 'Group 1'
      | sbobj.Groups.Signals.Name = 'Signal 1'
      | sbobj.Groups.Signals.XData = [0 0.18 0.3 0.45 1 2]
      | sbobj.Groups.Signals.YData = [0 0 1 1 1 1]
      | sbobj.Groups.TimeRange = [0 2]
  Signal 1 : Outport  Tag=STV Outport
  wires:
  Demux/1 -> Signal 1/1
  FromWs/1 -> Demux/1

== system RefBlocks/load torque and speed/load torque ==
  Demux : Demux  Tag=STV Demux  Outputs=1
      settings: DisplayOption=none
  FromWs : FromWorkspace  Tag=STV FromWs  VariableName=tuvar
      SigBuilderData=|
      | common.afterFinalStr = 'Extrapolate'
      | common.sampleTime = 0
      | dataSet.timeRange = [0 10]
      | dataSet.name = 'Group 1'
      | sbobj.Groups.Name = 'Group 1'
      | sbobj.Groups.Signals.Name = 'Signal 1'
      | sbobj.Groups.Signals.XData = [0 0.12 0.25 8.64 8.64 10]
      | sbobj.Groups.Signals.YData = [0 0 1 1 -0.98 -0.98]
  Signal 1 : Outport  Tag=STV Outport
  wires:
  FromWs/1 -> Demux/1
  Demux/1 -> Signal 1/1

== system RefBlocks/Inverse Flux Maps/Inverse Flux Maps /2D LUT ==
  Fdq : Inport
  dq Model : Subsystem  Variant=on
  idq : Outport
  T : Outport  Port=2
  wires:
  Fdq/1 -> dq Model/1(Fdq)
  dq Model/1(idq) -> idq/1
  dq Model/2(T) -> T/1

== system RefBlocks/Inverse Flux Maps/Inverse Flux Maps /3D LUTs ==
  Fdq : Inport
  theta_elt : Inport  Port=2
  Variant Subsystem : Subsystem  Variant=on
  idq : Outport
  T : Outport  Port=2
  wires:
  Fdq/1 -> Variant Subsystem/1(Fdq)
  Variant Subsystem/1(idq) -> idq/1
  Variant Subsystem/2(T) -> T/1
  theta_elt/1 -> Variant Subsystem/2(theta_elt)

== system RefBlocks/Inverter Model/Inverter Commands/Duty ==
  Dabc : Inport
  iABC : Inport  Port=2
  Demux : Demux  Outputs=3
  Gain : Gain  Gain=dT/Ts
  Mux14 : Mux  Inputs=6
  Sign : Signum
  Sum : Sum  Inputs=|+-
  X_d1 : Fcn  Expr=1-u(1)
  X_d12 : Fcn  Expr=1-u(1)
  X_d2 : Fcn  Expr=1-u(1)
  G : Outport  VectorParamsAs1DForOutWhenUnconnected=off
  wires:
  iABC/1 -> Sign/1
  Sign/1 -> Gain/1
  Demux/3 -> Mux14/5, X_d2/1
  X_d2/1 -> Mux14/6
  Demux/1 -> X_d12/1, Mux14/1
  Dabc/1 -> Sum/1
  Gain/1 -> Sum/2
  Sum/1 -> Demux/1
  Demux/2 -> Mux14/3, X_d1/1
  X_d1/1 -> Mux14/4
  X_d12/1 -> Mux14/2
  Mux14/1 -> G/1

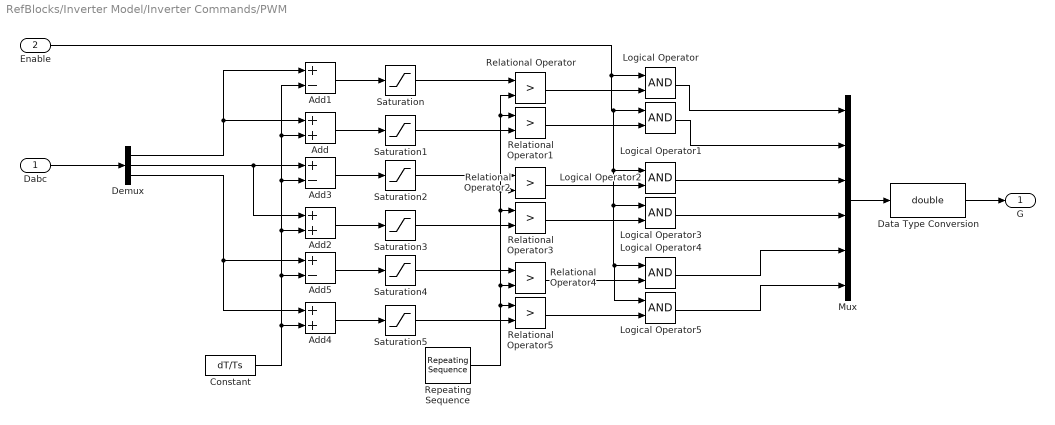
== system RefBlocks/Inverter Model/Inverter Commands/PWM ==
  Dabc : Inport
  Enable : Inport  Port=2
  Add : Sum
  Add1 : Sum  Inputs=+-
  Add2 : Sum
  Add3 : Sum  Inputs=+-
  Add4 : Sum
  Add5 : Sum  Inputs=+-
  Constant : Constant  Value=dT/Ts
  Data Type Conversion : DataTypeConversion  OutDataTypeStr=double
  Demux : Demux  Outputs=3
  Logical Operator{,1..5} (6 alike) : Logic  AllPortsSameDT=off  OutDataTypeStr=boolean
  Mux : Mux  Inputs=6
  Relational Operator{,1..5} (6 alike) : RelationalOperator  Operator=>  OutDataTypeStr=boolean  RndMeth=Simplest
  Repeating Sequence : simulink/Sources/Repeating Sequence  rep_seq_t=[0 Ts/2 Ts]  rep_seq_y=[0 1 0]
  Saturation{,1..5} (6 alike) : Saturate  UpperLimit=1  LowerLimit=0
  G : Outport
  wires:
  Demux/3 -> Add4/1, Add5/1
  Add4/1 -> Saturation5/1
  Relational Operator4/1 -> Logical Operator4/2
  Add/1 -> Saturation1/1
  Relational Operator/1 -> Logical Operator/2
  Enable/1 -> Logical Operator5/1, Logical Operator4/1, Logical Operator3/1, Logical Operator2/1, Logical Operator1/1, Logical Operator/1
  Add5/1 -> Saturation4/1
  Relational Operator3/1 -> Logical Operator3/2
  Add1/1 -> Saturation/1
  Constant/1 -> Add1/2, Add/2, Add3/2, Add2/2, Add5/2, Add4/2
  Demux/1 -> Add1/1, Add/1
  Saturation2/1 -> Relational Operator2/1
  Demux/2 -> Add3/1, Add2/1
  Relational Operator2/1 -> Logical Operator2/2
  Saturation5/1 -> Relational Operator5/2
  Relational Operator1/1 -> Logical Operator1/2
  Add3/1 -> Saturation2/1
  Add2/1 -> Saturation3/1
  Saturation/1 -> Relational Operator/1
  Saturation4/1 -> Relational Operator4/1
  Saturation1/1 -> Relational Operator1/2
  Relational Operator5/1 -> Logical Operator5/2
  Logical Operator/1 -> Mux/1
  Saturation3/1 -> Relational Operator3/2
  Logical Operator1/1 -> Mux/2
  Dabc/1 -> Demux/1
  Mux/1 -> Data Type Conversion/1
  Logical Operator2/1 -> Mux/3
  Logical Operator3/1 -> Mux/4
  Logical Operator4/1 -> Mux/5
  Logical Operator5/1 -> Mux/6
  Repeating Sequence/1 -> Relational Operator/2, Relational Operator1/1, Relational Operator2/2, Relational Operator3/1, Relational Operator4/2, Relational Operator5/1
  Data Type Conversion/1 -> G/1

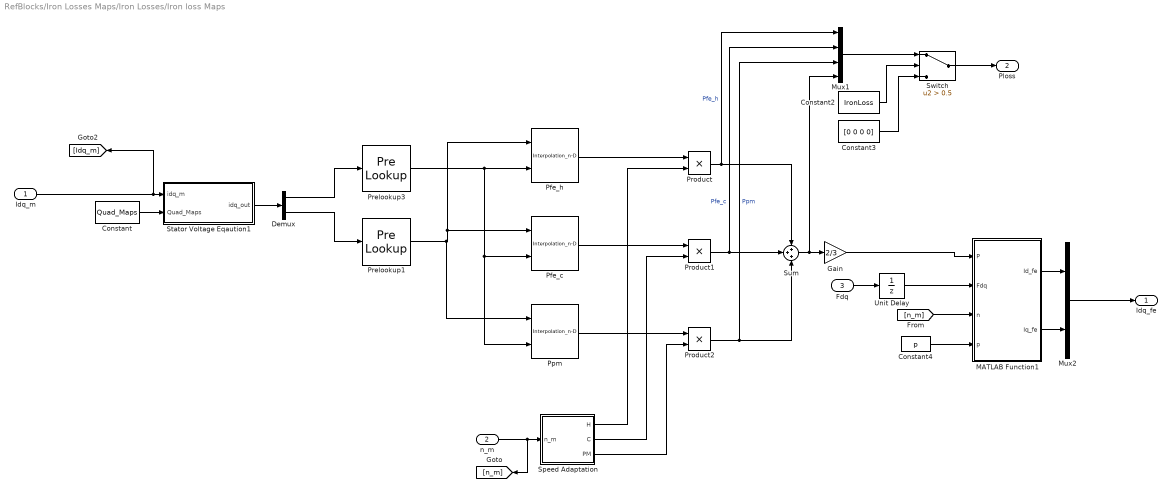
== system RefBlocks/Iron Losses Maps/Iron Losses/Iron loss Maps ==
  Idq_m : Inport
  n_m : Inport  Port=2
  Fdq : Inport  Port=3
  Constant : Constant  Value=Quad_Maps
  Constant2 : Constant  Value=IronLoss
  Constant3 : Constant  Value=[0 0 0 0]
  Constant4 : Constant  Value=p
  Demux : Demux  Outputs=2
  Gain : Gain  Gain=2/3
  MATLAB Function1 : MATLAB Function  TreatAsAtomicUnit=on
  Mux1 : Mux
  Mux2 : Mux  Inputs=2
  Pfe_c : Interpolation_n-D  Table=Pfe_c  RequireIndexFractionAsBus=on  InternalRulePriority=Speed
      settings: InputPortMap=u0,u1
  Pfe_h : Interpolation_n-D  Table=Pfe_h  RequireIndexFractionAsBus=on  InternalRulePriority=Speed
      settings: InputPortMap=u0,u1
  Ppm : Interpolation_n-D  Table=Ppm  RequireIndexFractionAsBus=on  InternalRulePriority=Speed
      settings: InputPortMap=u0,u1
  Prelookup1 : PreLookup  BreakpointsData=Iq_fe(:,1)  OutputSelection=Index and fraction as bus  ExtrapMethod=Linear
  Prelookup3 : PreLookup  BreakpointsData=Id_fe(1,:)  OutputSelection=Index and fraction as bus  ExtrapMethod=Linear
  Product : Product
  Product1 : Product
  Product2 : Product
  Speed Adaptation : Subsystem
  Stator Voltage Eqaution1 : MATLAB Function  TreatAsAtomicUnit=on
  Sum : Sum  Inputs=+++
  Switch : Switch  Criteria=u2 > Threshold  Threshold=0.5
  Unit Delay : UnitDelay  SampleTime=-1  HasFrameUpgradeWarning=on
  Idq_fe : Outport
  Ploss : Outport  Port=2
  wires:
  Product1/1 -> Mux1/2, Sum/2  "Pfe_c"
  Product2/1 -> Mux1/3, Sum/3  "Ppm"
  Pfe_h/1 -> Product/1
  Prelookup3/1 -> Ppm/2, Pfe_c/2, Pfe_h/2
  Speed Adaptation/1(H) -> Product/2
  n_m/1 -> Speed Adaptation/1(n_m), [n_m]
  Demux/1 -> Prelookup3/1
  Sum/1 -> Mux1/4, Gain/1
  Product/1 -> Sum/1, Mux1/1  "Pfe_h"
  Speed Adaptation/2(C) -> Product1/2
  Prelookup1/1 -> Ppm/1, Pfe_h/1, Pfe_c/1
  Pfe_c/1 -> Product1/1
  Ppm/1 -> Product2/1
  Demux/2 -> Prelookup1/1
  Speed Adaptation/3(PM) -> Product2/2
  Constant/1 -> Stator Voltage Eqaution1/2(Quad_Maps)
  Stator Voltage Eqaution1/1(idq_out) -> Demux/1
  Idq_m/1 -> [Idq_m], Stator Voltage Eqaution1/1(idq_m)
  Gain/1 -> MATLAB Function1/1(P)
  Fdq/1 -> Unit Delay/1
  [n_m] -> MATLAB Function1/3(n)
  Constant4/1 -> MATLAB Function1/4(p)
  MATLAB Function1/1(Id_fe) -> Mux2/1
  Mux2/1 -> Idq_fe/1
  Unit Delay/1 -> MATLAB Function1/2(Fdq)
  MATLAB Function1/2(Iq_fe) -> Mux2/2
  Mux1/1 -> Switch/1
  Constant2/1 -> Switch/2
  Switch/1 -> Ploss/1
  Constant3/1 -> Switch/3

== system RefBlocks/Inverse Flux Maps/Inverse Flux Maps /2D LUT/dq Model ==
  note: 1) Add Subsystem or Model blocks as valid variant choices.
      | 2) You cannot connect blocks at this level. At simulation, connectivity is automatically
      | determined, based on the active variant and port name matching.
  Fdq : Inport
  IPM : Subsystem  VariantControl=Quad_Maps==2
  PM-SyR : Subsystem  VariantControl=Quad_Maps==1
  SyR : Subsystem  VariantControl=Quad_Maps==0
  idq : Outport
  T : Outport  Port=2

== system RefBlocks/Inverse Flux Maps/Inverse Flux Maps /3D LUTs/Variant Subsystem ==
  note: 1) Add Subsystem or Model blocks as valid variant choices.
      | 2) You cannot connect blocks at this level. At simulation, connectivity is automatically
      | determined, based on the active variant and port name matching.
  Fdq : Inport
  theta_elt : Inport  Port=2
  IPM : Subsystem  VariantControl=Quad_Maps==2
  PM-SyR : Subsystem  VariantControl=Quad_Maps==1
  SyR : Subsystem  VariantControl=Quad_Maps==0
  idq : Outport
  T : Outport  Port=2

== system RefBlocks/Iron Losses Maps/Iron Losses/Iron loss Maps/Speed Adaptation ==
  n_m : Inport
  Constant : Constant  Value=n0
  Constant1 : Constant  Value=expC
  Constant2 : Constant  Value=expH
  Constant3 : Constant  Value=expPM
  Divide : Product  Inputs=*/
  Math Function : Math  Operator=pow  SignedPower=on  SaturateOnIntegerOverflow=on
  Math Function1 : Math  Operator=pow  SignedPower=on  SaturateOnIntegerOverflow=on
  Math Function2 : Math  Operator=pow  SignedPower=on  SaturateOnIntegerOverflow=on
  H : Outport
  C : Outport  Port=2
  PM : Outport  Port=3
  wires:
  Math Function2/1 -> PM/1
  Math Function/1 -> H/1
  Constant1/1 -> Math Function1/2
  Divide/1 -> Math Function/1, Math Function1/1, Math Function2/1
  Math Function1/1 -> C/1
  Constant/1 -> Divide/2
  Constant2/1 -> Math Function/2
  Constant3/1 -> Math Function2/2
  n_m/1 -> Divide/1

== system RefBlocks/Inverse Flux Maps/Inverse Flux Maps /2D LUT/dq Model/IPM ==
  Fdq : Inport
  1-D Lookup Table : Lookup_n-D  NumberOfTableDimensions=1  BreakpointsForDimension1=fD_vct_ref  Table=fQ_vct_max  InternalRulePriority=Speed  RndMeth=Simplest  InputSameDT=on
  Abs1 : Abs
  Bias : Bias  Bias=-fD_vct_ref(1)
  Constant : Constant  Value=fD_vct_ref(end)-fD_vct_ref(1)
  Demux : Demux  Outputs=2
  Divide : Product  Inputs=*/
  Divide1 : Product  Inputs=/*
  Id_pu : Lookup_n-D  BreakpointsForDimension1=fQ_pu_norm(:,1)  BreakpointsForDimension2=fD_pu_norm(1,:)  Table=iD_pu_norm  InternalRulePriority=Speed  RndMeth=Simplest  InputSameDT=on
      settings: InputPortMap=u0,u1
  Iq_pu : Lookup_n-D  BreakpointsForDimension1=fQ_pu_norm(:,1)  BreakpointsForDimension2=fD_pu_norm(1,:)  Table=iQ_pu_norm  InternalRulePriority=Speed  RndMeth=Simplest  InputSameDT=on
      settings: InputPortMap=u0,u1
  Mux : Mux  Inputs=2
  Product1 : Product
  Saturation : Saturate  UpperLimit=fD_vct_ref(end)  LowerLimit=fD_vct_ref(1)
  Saturation Dynamic : simulink/Discontinuities/Saturation Dynamic  OutMin=[]  OutMax=[]  OutDataTypeStr=Inherit: Same as second input  OutDataType=fixdt(1, 16)  OutScaling=2^-10  DoSatur=off
  Sign1 : Signum
  Torque calculation : Subsystem
  idq : Outport
  T : Outport  Port=2
  wires:
  Iq_pu/1 -> Product1/1
  Demux/2 -> Sign1/1, Abs1/1
  Sign1/1 -> Product1/2
  Fdq/1 -> Torque calculation/2(Fdq), Demux/1
  Mux/1 -> Torque calculation/1(Idq), idq/1
  Bias/1 -> Divide/1
  Product1/1 -> Mux/2  "iq_pu"
  Constant/1 -> Divide/2
  1-D Lookup Table/1 -> Divide1/1, Saturation Dynamic/1
  Torque calculation/1(Tm) -> T/1
  Saturation Dynamic/1 -> Divide1/2
  Abs1/1 -> Saturation Dynamic/3, Saturation Dynamic/2
  Divide1/1 -> Id_pu/1, Iq_pu/1
  Demux/1 -> Saturation/1
  Divide/1 -> Iq_pu/2, Id_pu/2
  Saturation/1 -> Bias/1, 1-D Lookup Table/1
  Id_pu/1 -> Mux/1  "iq_pu"

== system RefBlocks/Inverse Flux Maps/Inverse Flux Maps /2D LUT/dq Model/PM-SyR ==
  Fdq : Inport
  1-D Lookup Table : Lookup_n-D  NumberOfTableDimensions=1  BreakpointsForDimension1=fQ_vct_ref  Table=fD_vct_max  InternalRulePriority=Speed  RndMeth=Simplest  InputSameDT=on
  Abs : Abs
  Bias : Bias  Bias=-fQ_vct_ref(1)
  Constant : Constant  Value=fQ_vct_ref(end)-fQ_vct_ref(1)
  Demux : Demux  Outputs=2
  Divide : Product  Inputs=*/
  Divide1 : Product  Inputs=/*
  Id_pu : Lookup_n-D  BreakpointsForDimension1=fQ_pu_norm(:,1)  BreakpointsForDimension2=fD_pu_norm(1,:)  Table=iD_pu_norm  InternalRulePriority=Speed  RndMeth=Simplest  InputSameDT=on
      settings: InputPortMap=u0,u1
  Iq_pu : Lookup_n-D  BreakpointsForDimension1=fQ_pu_norm(:,1)  BreakpointsForDimension2=fD_pu_norm(1,:)  Table=iQ_pu_norm  InternalRulePriority=Speed  RndMeth=Simplest  InputSameDT=on
      settings: InputPortMap=u0,u1
  Mux : Mux  Inputs=2
  Product2 : Product
  Saturation : Saturate  UpperLimit=fQ_vct_ref(end)  LowerLimit=fQ_vct_ref(1)
  Saturation Dynamic : simulink/Discontinuities/Saturation Dynamic  OutMin=[]  OutMax=[]  OutDataTypeStr=Inherit: Same as second input  OutDataType=fixdt(1, 16)  OutScaling=2^-10  DoSatur=off
  Sign2 : Signum
  Torque calculation : Subsystem
  idq : Outport
  T : Outport  Port=2
  wires:
  Torque calculation/1(Tm) -> T/1
  Saturation/1 -> Bias/1, 1-D Lookup Table/1
  Bias/1 -> Divide/1
  Saturation Dynamic/1 -> Divide1/2
  Iq_pu/1 -> Mux/2  "iq_pu"
  1-D Lookup Table/1 -> Divide1/1, Saturation Dynamic/1
  Sign2/1 -> Product2/1
  Fdq/1 -> Torque calculation/2(Fdq), Demux/1
  Id_pu/1 -> Product2/2
  Product2/1 -> Mux/1  "id_pu"
  Mux/1 -> idq/1, Torque calculation/1(Idq)
  Constant/1 -> Divide/2
  Abs/1 -> Saturation Dynamic/3, Saturation Dynamic/2
  Demux/2 -> Saturation/1
  Demux/1 -> Sign2/1, Abs/1
  Divide1/1 -> Id_pu/2, Iq_pu/2
  Divide/1 -> Iq_pu/1, Id_pu/1

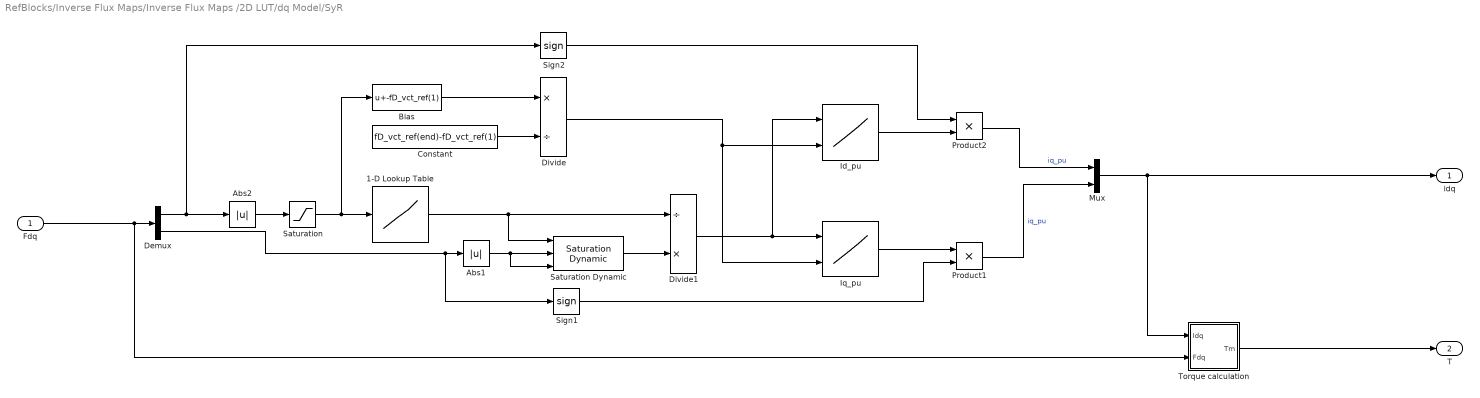
== system RefBlocks/Inverse Flux Maps/Inverse Flux Maps /2D LUT/dq Model/SyR ==
  Fdq : Inport
  1-D Lookup Table : Lookup_n-D  NumberOfTableDimensions=1  BreakpointsForDimension1=fD_vct_ref  Table=fQ_vct_max  InternalRulePriority=Speed  RndMeth=Simplest  InputSameDT=on
  Abs1 : Abs
  Abs2 : Abs
  Bias : Bias  Bias=-fD_vct_ref(1)
  Constant : Constant  Value=fD_vct_ref(end)-fD_vct_ref(1)
  Demux : Demux  Outputs=2
  Divide : Product  Inputs=*/
  Divide1 : Product  Inputs=/*
  Id_pu : Lookup_n-D  BreakpointsForDimension1=fQ_pu_norm(:,1)  BreakpointsForDimension2=fD_pu_norm(1,:)  Table=iD_pu_norm  InternalRulePriority=Speed  RndMeth=Simplest  InputSameDT=on
      settings: InputPortMap=u0,u1
  Iq_pu : Lookup_n-D  BreakpointsForDimension1=fQ_pu_norm(:,1)  BreakpointsForDimension2=fD_pu_norm(1,:)  Table=iQ_pu_norm  InternalRulePriority=Speed  RndMeth=Simplest  InputSameDT=on
      settings: InputPortMap=u0,u1
  Mux : Mux  Inputs=2
  Product1 : Product
  Product2 : Product
  Saturation : Saturate  UpperLimit=fD_vct_ref(end)  LowerLimit=fD_vct_ref(1)
  Saturation Dynamic : simulink/Discontinuities/Saturation Dynamic  OutMin=[]  OutMax=[]  OutDataTypeStr=Inherit: Same as second input  OutDataType=fixdt(1, 16)  OutScaling=2^-10  DoSatur=off
  Sign1 : Signum
  Sign2 : Signum
  Torque calculation : Subsystem
  idq : Outport
  T : Outport  Port=2
  wires:
  Fdq/1 -> Torque calculation/2(Fdq), Demux/1
  Mux/1 -> Torque calculation/1(Idq), idq/1
  Product1/1 -> Mux/2  "iq_pu"
  Constant/1 -> Divide/2
  Bias/1 -> Divide/1
  Divide/1 -> Iq_pu/2, Id_pu/2
  Demux/2 -> Sign1/1, Abs1/1
  Saturation/1 -> Bias/1, 1-D Lookup Table/1
  Divide1/1 -> Id_pu/1, Iq_pu/1
  Demux/1 -> Abs2/1, Sign2/1
  Abs1/1 -> Saturation Dynamic/3, Saturation Dynamic/2
  Sign1/1 -> Product1/2
  Iq_pu/1 -> Product1/1
  1-D Lookup Table/1 -> Divide1/1, Saturation Dynamic/1
  Saturation Dynamic/1 -> Divide1/2
  Id_pu/1 -> Product2/2
  Product2/1 -> Mux/1  "iq_pu"
  Abs2/1 -> Saturation/1
  Sign2/1 -> Product2/1
  Torque calculation/1(Tm) -> T/1

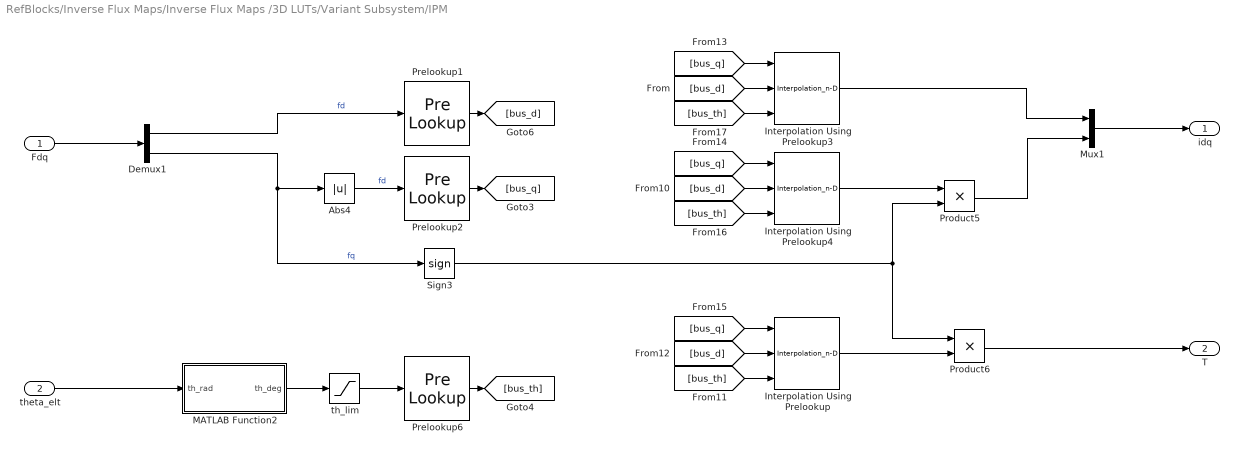
== system RefBlocks/Inverse Flux Maps/Inverse Flux Maps /3D LUTs/Variant Subsystem/IPM ==
  Fdq : Inport
  theta_elt : Inport  Port=2
  Abs4 : Abs
  Demux1 : Demux  Outputs=2
  Interpolation Using Prelookup : Interpolation_n-D  NumberOfTableDimensions=3  Table=T_dqt  LookupTableObject=T_th  RequireIndexFractionAsBus=on  InternalRulePriority=Speed
      settings: InputPortMap=u0,u1,u2
  Interpolation Using Prelookup3 : Interpolation_n-D  NumberOfTableDimensions=3  Table=Id_dqt  RequireIndexFractionAsBus=on  InternalRulePriority=Speed
      settings: InputPortMap=u0,u1,u2
  Interpolation Using Prelookup4 : Interpolation_n-D  NumberOfTableDimensions=3  Table=Iq_dqt  RequireIndexFractionAsBus=on  InternalRulePriority=Speed
      settings: InputPortMap=u0,u1,u2
  MATLAB Function2 : MATLAB Function  TreatAsAtomicUnit=on
  Mux1 : Mux  Inputs=2
  Prelookup1 : PreLookup  BreakpointsData=Fd_v  OutputSelection=Index and fraction as bus  ExtrapMethod=Linear
  Prelookup2 : PreLookup  BreakpointsData=Fq_v  OutputSelection=Index and fraction as bus  ExtrapMethod=Linear
  Prelookup6 : PreLookup  BreakpointsData=th_v  OutputSelection=Index and fraction as bus  ExtrapMethod=Linear
  Product5 : Product
  Product6 : Product
  Sign3 : Signum
  th_lim : Saturate  UpperLimit=th_max  LowerLimit=th_min  ZeroCross=off
  idq : Outport
  T : Outport  Port=2
  wires:
  theta_elt/1 -> MATLAB Function2/1(th_rad)
  Sign3/1 -> Product6/1, Product5/2
  Interpolation Using Prelookup3/1 -> Mux1/1
  Product5/1 -> Mux1/2
  Product6/1 -> T/1
  Interpolation Using Prelookup4/1 -> Product5/1
  Abs4/1 -> Prelookup2/1  "fd"
  MATLAB Function2/1(th_deg) -> th_lim/1
  [bus_d] -> Interpolation Using Prelookup3/2
  [bus_d] -> Interpolation Using Prelookup4/2
  Prelookup1/1 -> [bus_d]
  [bus_q] -> Interpolation Using Prelookup/1
  Demux1/2 -> Sign3/1, Abs4/1  "fq"
  [bus_th] -> Interpolation Using Prelookup/3
  [bus_q] -> Interpolation Using Prelookup4/1
  [bus_d] -> Interpolation Using Prelookup/2
  [bus_q] -> Interpolation Using Prelookup3/1
  [bus_th] -> Interpolation Using Prelookup4/3
  Demux1/1 -> Prelookup1/1  "fd"
  th_lim/1 -> Prelookup6/1
  Prelookup6/1 -> [bus_th]
  [bus_th] -> Interpolation Using Prelookup3/3
  Prelookup2/1 -> [bus_q]
  Mux1/1 -> idq/1
  Fdq/1 -> Demux1/1
  Interpolation Using Prelookup/1 -> Product6/2

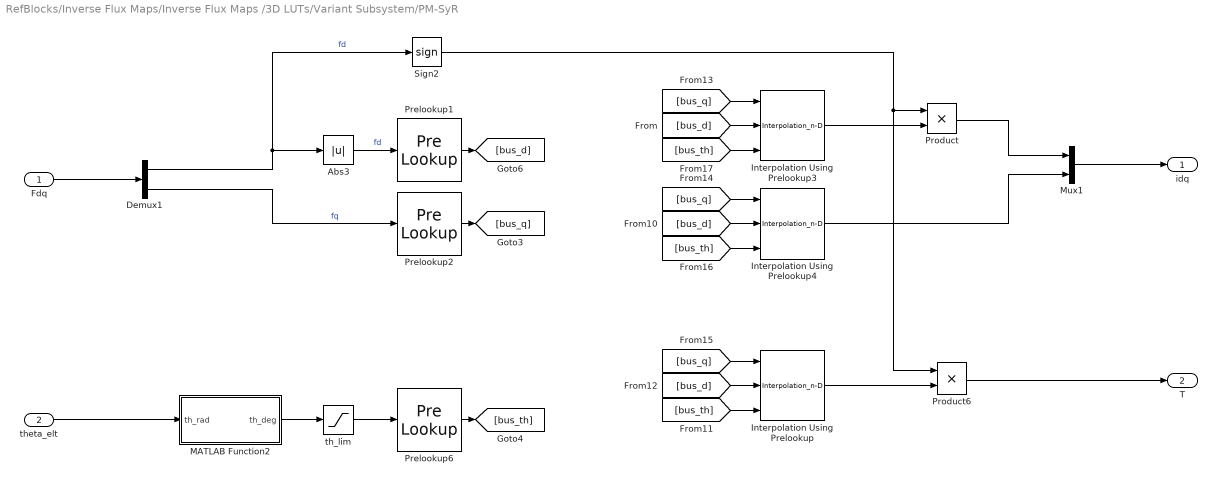
== system RefBlocks/Inverse Flux Maps/Inverse Flux Maps /3D LUTs/Variant Subsystem/PM-SyR ==
  Fdq : Inport
  theta_elt : Inport  Port=2
  Abs3 : Abs
  Demux1 : Demux  Outputs=2
  Interpolation Using Prelookup : Interpolation_n-D  NumberOfTableDimensions=3  Table=T_dqt  LookupTableObject=T_th  RequireIndexFractionAsBus=on  InternalRulePriority=Speed
      settings: InputPortMap=u0,u1,u2
  Interpolation Using Prelookup3 : Interpolation_n-D  NumberOfTableDimensions=3  Table=Id_dqt  RequireIndexFractionAsBus=on  InternalRulePriority=Speed
      settings: InputPortMap=u0,u1,u2
  Interpolation Using Prelookup4 : Interpolation_n-D  NumberOfTableDimensions=3  Table=Iq_dqt  RequireIndexFractionAsBus=on  InternalRulePriority=Speed
      settings: InputPortMap=u0,u1,u2
  MATLAB Function2 : MATLAB Function  TreatAsAtomicUnit=on
  Mux1 : Mux  Inputs=2
  Prelookup1 : PreLookup  BreakpointsData=Fd_v  OutputSelection=Index and fraction as bus  ExtrapMethod=Linear
  Prelookup2 : PreLookup  BreakpointsData=Fq_v  OutputSelection=Index and fraction as bus  ExtrapMethod=Linear
  Prelookup6 : PreLookup  BreakpointsData=th_v  OutputSelection=Index and fraction as bus  ExtrapMethod=Linear
  Product : Product
  Product6 : Product
  Sign2 : Signum
  th_lim : Saturate  UpperLimit=th_max  LowerLimit=th_min  ZeroCross=off
  idq : Outport
  T : Outport  Port=2
  wires:
  Sign2/1 -> Product6/1, Product/1
  Interpolation Using Prelookup3/1 -> Product/2
  ? -> ?
  theta_elt/1 -> MATLAB Function2/1(th_rad)
  Product/1 -> Mux1/1
  Interpolation Using Prelookup4/1 -> Mux1/2
  Product6/1 -> T/1
  Abs3/1 -> Prelookup1/1  "fd"
  MATLAB Function2/1(th_deg) -> th_lim/1
  [bus_d] -> Interpolation Using Prelookup3/2
  [bus_d] -> Interpolation Using Prelookup4/2
  Prelookup1/1 -> [bus_d]
  [bus_q] -> Interpolation Using Prelookup/1
  Demux1/2 -> Prelookup2/1  "fq"
  [bus_th] -> Interpolation Using Prelookup/3
  [bus_q] -> Interpolation Using Prelookup4/1
  [bus_d] -> Interpolation Using Prelookup/2
  [bus_q] -> Interpolation Using Prelookup3/1
  [bus_th] -> Interpolation Using Prelookup4/3
  Demux1/1 -> Sign2/1, Abs3/1  "fd"
  th_lim/1 -> Prelookup6/1
  Prelookup6/1 -> [bus_th]
  [bus_th] -> Interpolation Using Prelookup3/3
  Prelookup2/1 -> [bus_q]
  Mux1/1 -> idq/1
  Fdq/1 -> Demux1/1
  Interpolation Using Prelookup/1 -> Product6/2
